simulink model "modello_prova_kalman_17_03"  (R2020b)
settings: Solver=VariableStepAuto  StartTime=0.0  StopTime=800  RelTol=1e-3
values from neighbouring files (symbols this model uses):
  bias = [baccxINI_new,baccyINI_new,bacczINI_new,bpINI_new,bqINI_new,brINI_new]    [Loader_HIL.m]
  Sensor_Offsets = [0,0,0]    [Loader_HIL.m]
  UP = 2    [Loader_HIL.m]
  vd_ini = 0    [Loader_HIL.m]
undefined symbols (not defined in the file or in its folder): Q1B, R1B, t_AP
libraries: simulink_extras x6, aerosimlib x2, cstblocks x1, dspsigops x1
settings Model: Creator=User  LastModifiedBy=SUSANNA

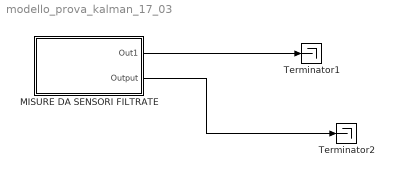
== system modello_prova_kalman_17_03 ==
  MISURE DA SENSORI FILTRATE : Subsystem
  Terminator1 : Terminator
  Terminator2 : Terminator
  wires:
  MISURE DA SENSORI FILTRATE/1(Out1) -> Terminator1/1
  MISURE DA SENSORI FILTRATE/2(Output) -> Terminator2/1

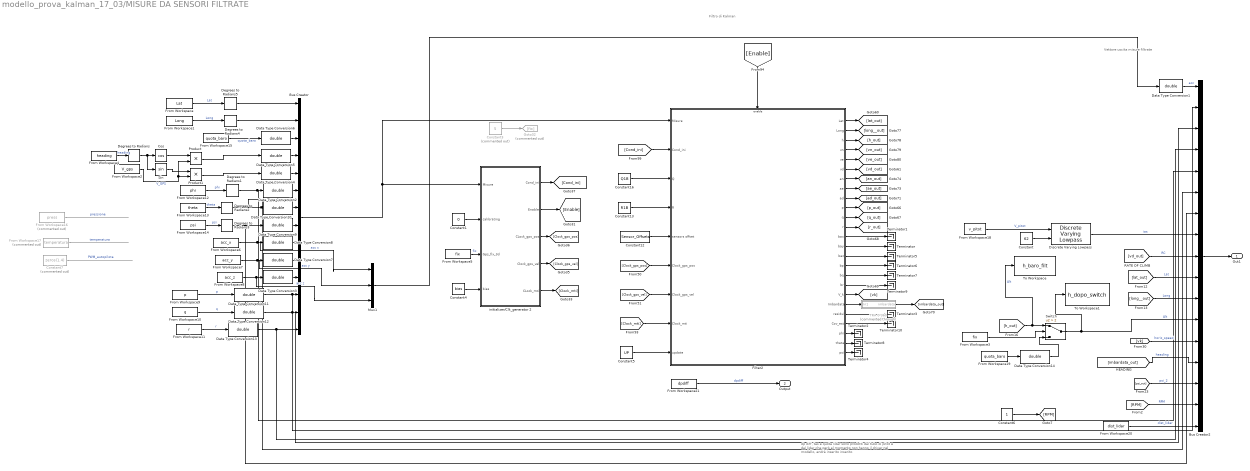
== system modello_prova_kalman_17_03/MISURE DA SENSORI FILTRATE ==
  note: dp diff, tas e quota lidar
      |  sono prodotti dal tubo di pitot e dal lidar che però al momento non hanno il driver nel modello, andrà inserito inserito
  note: Vettore uscita misure filtrate
  note: Filtro di Kalman
  Bus Creator : BusCreator  Inputs=14
  Bus Creator2 : BusCreator  Inputs=17
  Constant : Constant  Value=62
  Constant1 : Constant  Value=0
  Constant12 : Constant  Value=Sensor_Offsets
  Constant13 : Constant  Value=R1B
  Constant16 : Constant  Value=Q1B
  Constant3 : Constant  Commented=on  Value=5
  Constant4 : Constant  Value=bias
  Constant5 : Constant  Value=UP
  Constant6 : Constant
  Constant7 : Constant  Commented=on  Value=zeros(1,4)
  Cos : Trigonometry  Operator=cos
  Data Type Conversion{1..14} (14 alike) : DataTypeConversion  OutDataTypeStr=double
  Degrees to Radians{,1..5} (6 alike) : simulink_extras/Transformations/Degrees to Radians
  Discrete Varying Lowpass : cstblocks/Linear Parameter Varying/Discrete Varying Lowpass  N=1  w0=0  Ts=t_AP
      settings: SourceProductBaseCode=CT
  Filter2 : Subsystem
  From Workspace : FromWorkspace  VariableName=Lat  SampleTime=0.02
  From Workspace1 : FromWorkspace  VariableName=Long  SampleTime=0.02
  From Workspace10 : FromWorkspace  VariableName=q  SampleTime=0.02
  From Workspace11 : FromWorkspace  VariableName=r  SampleTime=0.02
  From Workspace12 : FromWorkspace  VariableName=phi  SampleTime=0.02
  From Workspace13 : FromWorkspace  VariableName=theta  SampleTime=0.02
  From Workspace14 : FromWorkspace  VariableName=psi  SampleTime=0.02
  From Workspace15 : FromWorkspace  VariableName=quota_baro
  From Workspace16 : FromWorkspace  Commented=on  VariableName=press
  From Workspace17 : FromWorkspace  Commented=on  VariableName=temperatura
  From Workspace18 : FromWorkspace  VariableName=v_pitot  SampleTime=0.02
  From Workspace19 : FromWorkspace  VariableName=quota_baro  SampleTime=0.02
  From Workspace2 : FromWorkspace  VariableName=V_gps  SampleTime=0.02
  From Workspace20 : FromWorkspace  VariableName=dist_lidar  SampleTime=0.02
  From Workspace21 : FromWorkspace  VariableName=dpdiff
  From Workspace3 : FromWorkspace  VariableName=fix  SampleTime=0.02
  From Workspace4 : FromWorkspace  VariableName=heading  SampleTime=0.02
  From Workspace5 : FromWorkspace  VariableName=fix
  From Workspace6 : FromWorkspace  VariableName=acc_x  SampleTime=0.02
  From Workspace7 : FromWorkspace  VariableName=acc_y  SampleTime=0.02
  From Workspace8 : FromWorkspace  VariableName=acc_z  SampleTime=0.02
  From Workspace9 : FromWorkspace  VariableName=p  SampleTime=0.02
  Goto32 : Goto  Commented=on  GotoTag=fix
  Mux1 : Mux  Inputs=3
  Product : Product
  Product1 : Product
  Sin : Trigonometry
  Switch : Switch  Criteria=u2 > Threshold  Threshold=2
  TRA 0-360 : Subsystem  Commented=through
  Terminator{,1..10} (11 alike) : Terminator
  To Workspace : ToWorkspace  VariableName=h_baro_filt  SaveFormat=Timeseries  SampleTime=-1
  To Workspace1 : ToWorkspace  VariableName=h_dopo_switch  SaveFormat=Timeseries  SampleTime=-1
  initializer/Clk_generator 2 : Subsystem
  Out1 : Outport  VectorParamsAs1DForOutWhenUnconnected=off
  Output : Outport  Port=2
  wires:
  From Workspace11/1 -> Data Type Conversion13/1  "r"
  [vd_out] -> Bus Creator2/9  "RC"
  From Workspace12/1 -> Degrees to Radians1/1  "phi"
  From Workspace9/1 -> Data Type Conversion11/1  "p"
  [vk] -> Bus Creator2/13  "horiz_speed"
  [imbardata_out] -> Bus Creator2/14  "heading"
  From Workspace10/1 -> Data Type Conversion12/1  "q"
  From Workspace13/1 -> Degrees to Radians2/1  "theta"
  Bus Creator2/1 -> Out1/1
  Discrete Varying Lowpass/1 -> Bus Creator2/8  "ias"
  [RPM] -> Bus Creator2/16  "RPM"
  Data Type Conversion1/1 -> Bus Creator2/1  "acc"
  Mux1/1 -> Data Type Conversion1/1
  From Workspace14/1 -> Degrees to Radians3/1  "psi"
  [long__out] -> Bus Creator2/11  "Long"
  [h_out] -> To Workspace/1, Switch/1  "Alt"
  [lat_out] -> Bus Creator2/10  "Lat"
  initializer/Clk_generator 2/5(CLock_mti) -> [Clock_mti]
  Constant3/1 -> Goto32/1
  initializer/Clk_generator 2/2(Enable) -> [Enable]
  Constant1/1 -> initializer/Clk_generator 2/2(calibrating)
  initializer/Clk_generator 2/3(CLock_gps_pos) -> [Clock_gps_pos]
  Filter2/3(h) -> [h_out]
  Constant4/1 -> initializer/Clk_generator 2/4(bias)
  Filter2/25(psi) -> Terminator4/1
  Filter2/6(vd) -> [vd_out]
  Constant13/1 -> Filter2/4(R)
  Filter2/10(p) -> [p_out]
  Filter2/18(br) -> Terminator9/1
  Filter2/23(phi) -> Terminator2/1
  Filter2/14(bay) -> Terminator/1
  [Cond_ini] -> Filter2/2(Cond_ini)
  Filter2/7(an) -> [an_out]
  Filter2/12(r) -> [r_out]
  initializer/Clk_generator 2/1(Cond_ini) -> [Cond_ini]
  Filter2/24(theta) -> Terminator8/1
  Filter2/11(q) -> [q_out]
  initializer/Clk_generator 2/4("Clock_gps_vel ") -> [Clock_gps_vel]
  Bus Creator/1 -> initializer/Clk_generator 2/1(Misure), Filter2/1(Misure)
  Filter2/2(Long) -> [long__out]
  Filter2/8(ae) -> [ae_out]
  Filter2/16(bp) -> Terminator6/1
  Filter2/9(ad) -> [ad_out]
  Filter2/4(vn) -> [vn_out]
  Constant16/1 -> Filter2/3(Q)
  Filter2/22(Cov_est) -> Terminator10/1
  Filter2/17(bq) -> Terminator7/1
  Filter2/21(residui) -> Terminator3/1
  [Clock_gps_vel] -> Filter2/7(Clock_gps_vel)
  Filter2/1(Lat) -> [lat_out]
  Filter2/15(baz) -> Terminator5/1
  [Enable] -> Filter2/Enable
  Filter2/19(V_k) -> [vk]
  Filter2/20(Imbardata) -> TRA 0-360/1(In1)
  Constant12/1 -> Filter2/5(sensors offset)
  Filter2/13(bax) -> Terminator1/1
  Filter2/5(ve) -> [ve_out]
  Constant5/1 -> Filter2/9(update)
  [Clock_gps_pos] -> Filter2/6(Clock_gps_pos)
  TRA 0-360/1(imbardata) -> [imbardata_out]
  [Clock_mti] -> Filter2/8(Clock_mti)
  Constant/1 -> Discrete Varying Lowpass/2
  Constant6/1 -> [RPM]
  [psi_out] -> Bus Creator2/15  "psi_2"
  From Workspace3/1 -> Switch/2
  From Workspace19/1 -> Data Type Conversion14/1
  Switch/1 -> To Workspace1/1, Bus Creator2/12  "Alt"
  From Workspace17/1 -> ?  "temperatura"
  From Workspace20/1 -> Bus Creator2/17  "dist_lidar"
  From Workspace/1 -> Degrees to Radians5/1  "Lat"
  From Workspace1/1 -> Degrees to Radians4/1  "Long"
  From Workspace18/1 -> Discrete Varying Lowpass/1  "V_pitot"
  From Workspace6/1 -> Mux1/1, Data Type Conversion8/1  "acc x"
  From Workspace8/1 -> Data Type Conversion3/1, Mux1/3  "acc z"
  From Workspace15/1 -> Data Type Conversion6/1  "quota_baro"
  Constant7/1 -> ?  "PWM_autopilota"
  From Workspace16/1 -> ?  "pressione"
  From Workspace21/1 -> Output/1  "dpdiff"
  From Workspace4/1 -> Degrees to Radians/1  "heading"
  From Workspace2/1 -> Product1/2, Product/2  "V_GPS"
  Sin/1 -> Product1/1
  Cos/1 -> Product/1
  Product/1 -> Data Type Conversion5/1
  Product1/1 -> Data Type Conversion4/1
  From Workspace7/1 -> Data Type Conversion7/1, Mux1/2  "acc y"
  From Workspace5/1 -> initializer/Clk_generator 2/3(Gps_fix_3d)  "fix"
  Degrees to Radians/1 -> Sin/1, Cos/1
  Degrees to Radians1/1 -> Bus Creator2/5, Data Type Conversion2/1
  Degrees to Radians2/1 -> Data Type Conversion10/1, Bus Creator2/6
  Degrees to Radians3/1 -> Bus Creator2/7, Data Type Conversion9/1
  Degrees to Radians4/1 -> Bus Creator/2
  Degrees to Radians5/1 -> Bus Creator/1
  Data Type Conversion6/1 -> Bus Creator/3
  Data Type Conversion5/1 -> Bus Creator/4
  Data Type Conversion4/1 -> Bus Creator/5
  Data Type Conversion2/1 -> Bus Creator/6
  Data Type Conversion10/1 -> Bus Creator/7
  Data Type Conversion9/1 -> Bus Creator/8
  Data Type Conversion8/1 -> Bus Creator/9
  Data Type Conversion7/1 -> Bus Creator/10
  Data Type Conversion3/1 -> Bus Creator/11
  Data Type Conversion11/1 -> Bus Creator2/2, Bus Creator/12
  Data Type Conversion12/1 -> Bus Creator2/3, Bus Creator/13
  Data Type Conversion13/1 -> Bus Creator2/4, Bus Creator/14
  Data Type Conversion14/1 -> Switch/3

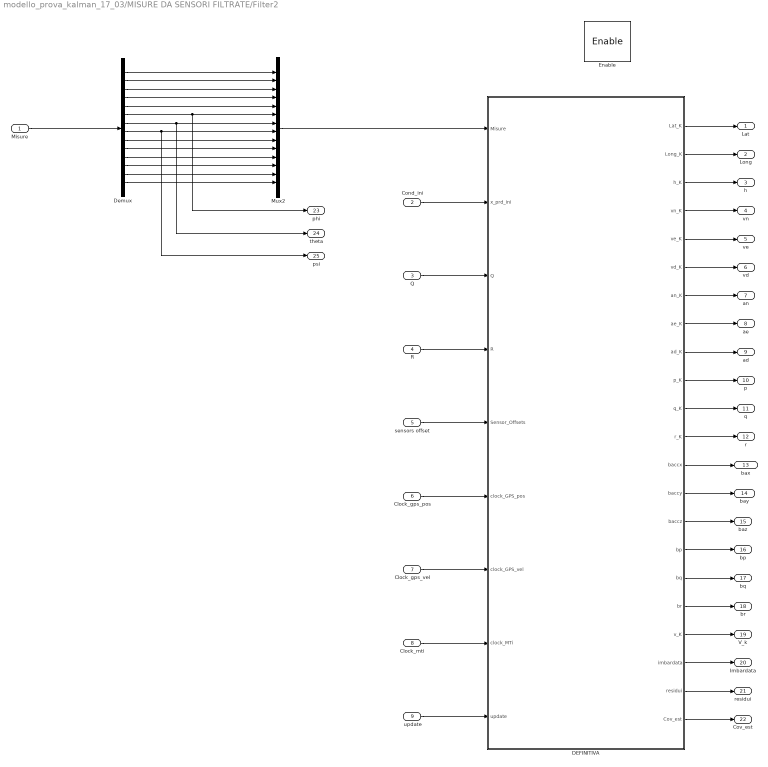
== system modello_prova_kalman_17_03/MISURE DA SENSORI FILTRATE/Filter2 ==
  Misure : Inport
  Cond_ini : Inport  Port=2
  Q : Inport  Port=3
  R : Inport  Port=4
  sensors offset : Inport  Port=5
  Clock_gps_pos : Inport  Port=6
  Clock_gps_vel : Inport  Port=7
  Clock_mti : Inport  Port=8
  update : Inport  Port=9
  Enable : EnablePort
  DEFINITIVA : MATLAB Function  TreatAsAtomicUnit=on
  Demux : Demux  Outputs=14
  Mux2 : Mux  Inputs=14
  Lat : Outport  VectorParamsAs1DForOutWhenUnconnected=off
  Long : Outport  Port=2  VectorParamsAs1DForOutWhenUnconnected=off
  h : Outport  Port=3  VectorParamsAs1DForOutWhenUnconnected=off
  vn : Outport  Port=4  VectorParamsAs1DForOutWhenUnconnected=off
  ve : Outport  Port=5  VectorParamsAs1DForOutWhenUnconnected=off
  vd : Outport  Port=6  VectorParamsAs1DForOutWhenUnconnected=off
  an : Outport  Port=7  VectorParamsAs1DForOutWhenUnconnected=off
  ae : Outport  Port=8  VectorParamsAs1DForOutWhenUnconnected=off
  ad : Outport  Port=9  VectorParamsAs1DForOutWhenUnconnected=off
  p : Outport  Port=10  VectorParamsAs1DForOutWhenUnconnected=off
  q : Outport  Port=11  VectorParamsAs1DForOutWhenUnconnected=off
  r : Outport  Port=12  VectorParamsAs1DForOutWhenUnconnected=off
  bax : Outport  Port=13  VectorParamsAs1DForOutWhenUnconnected=off
  bay : Outport  Port=14  VectorParamsAs1DForOutWhenUnconnected=off
  baz : Outport  Port=15  VectorParamsAs1DForOutWhenUnconnected=off
  bp : Outport  Port=16  VectorParamsAs1DForOutWhenUnconnected=off
  bq : Outport  Port=17  VectorParamsAs1DForOutWhenUnconnected=off
  br : Outport  Port=18  VectorParamsAs1DForOutWhenUnconnected=off
  V_k : Outport  Port=19  VectorParamsAs1DForOutWhenUnconnected=off
  Imbardata : Outport  Port=20  VectorParamsAs1DForOutWhenUnconnected=off
  residui : Outport  Port=21  VectorParamsAs1DForOutWhenUnconnected=off
  Cov_est : Outport  Port=22  VectorParamsAs1DForOutWhenUnconnected=off
  phi : Outport  Port=23  VectorParamsAs1DForOutWhenUnconnected=off
  theta : Outport  Port=24  VectorParamsAs1DForOutWhenUnconnected=off
  psi : Outport  Port=25  VectorParamsAs1DForOutWhenUnconnected=off
  wires:
  Misure/1 -> Demux/1
  Demux/10 -> Mux2/10
  Demux/13 -> Mux2/13
  Demux/11 -> Mux2/11
  Demux/4 -> Mux2/4
  Demux/14 -> Mux2/14
  Demux/7 -> theta/1, Mux2/7
  Demux/12 -> Mux2/12
  Demux/6 -> phi/1, Mux2/6
  Demux/5 -> Mux2/5
  Demux/9 -> Mux2/9
  Demux/8 -> psi/1, Mux2/8
  Demux/3 -> Mux2/3
  DEFINITIVA/8(ae_K) -> ae/1
  DEFINITIVA/7(an_K) -> an/1
  DEFINITIVA/11(q_K) -> q/1
  DEFINITIVA/2(Long_K) -> Long/1
  DEFINITIVA/3(h_K) -> h/1
  DEFINITIVA/10(p_K) -> p/1
  DEFINITIVA/6(vd_K) -> vd/1
  DEFINITIVA/13(baccx) -> bax/1
  DEFINITIVA/20(imbardata) -> Imbardata/1
  DEFINITIVA/19(v_K) -> V_k/1
  DEFINITIVA/18(br) -> br/1
  DEFINITIVA/4(vn_K) -> vn/1
  DEFINITIVA/16(bp) -> bp/1
  DEFINITIVA/21(residui) -> residui/1
  DEFINITIVA/17(bq) -> bq/1
  DEFINITIVA/5(ve_K) -> ve/1
  DEFINITIVA/12(r_K) -> r/1
  DEFINITIVA/1(Lat_K) -> Lat/1
  DEFINITIVA/22(Cov_est) -> Cov_est/1
  DEFINITIVA/15(baccz) -> baz/1
  DEFINITIVA/14(baccy) -> bay/1
  DEFINITIVA/9(ad_K) -> ad/1
  Mux2/1 -> DEFINITIVA/1(Misure)
  Cond_ini/1 -> DEFINITIVA/2(x_prd_ini)
  Q/1 -> DEFINITIVA/3(Q)
  R/1 -> DEFINITIVA/4(R)
  sensors offset/1 -> DEFINITIVA/5(Sensor_Offsets)
  Clock_gps_pos/1 -> DEFINITIVA/6(clock_GPS_pos)
  Clock_gps_vel/1 -> DEFINITIVA/7(clock_GPS_vel)
  Clock_mti/1 -> DEFINITIVA/8(clock_MTi)
  update/1 -> DEFINITIVA/9(update)
  Demux/2 -> Mux2/2
  Demux/1 -> Mux2/1

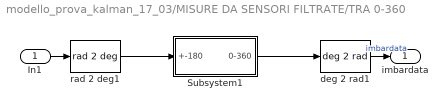
== system modello_prova_kalman_17_03/MISURE DA SENSORI FILTRATE/TRA 0-360 ==
  In1 : Inport
  Subsystem1 : Subsystem
  deg 2 rad1 : aerosimlib/Unit Conversion/Angular position/deg 2 rad
      settings: SourceProductName=AeroSim Blockset
  rad 2 deg1 : aerosimlib/Unit Conversion/Angular position/rad 2 deg
      settings: SourceProductName=AeroSim Blockset
  imbardata : Outport  VectorParamsAs1DForOutWhenUnconnected=off
  wires:
  deg 2 rad1/1 -> imbardata/1  "imbardata"
  rad 2 deg1/1 -> Subsystem1/1(+-180)
  In1/1 -> rad 2 deg1/1
  Subsystem1/1(0-360) -> deg 2 rad1/1

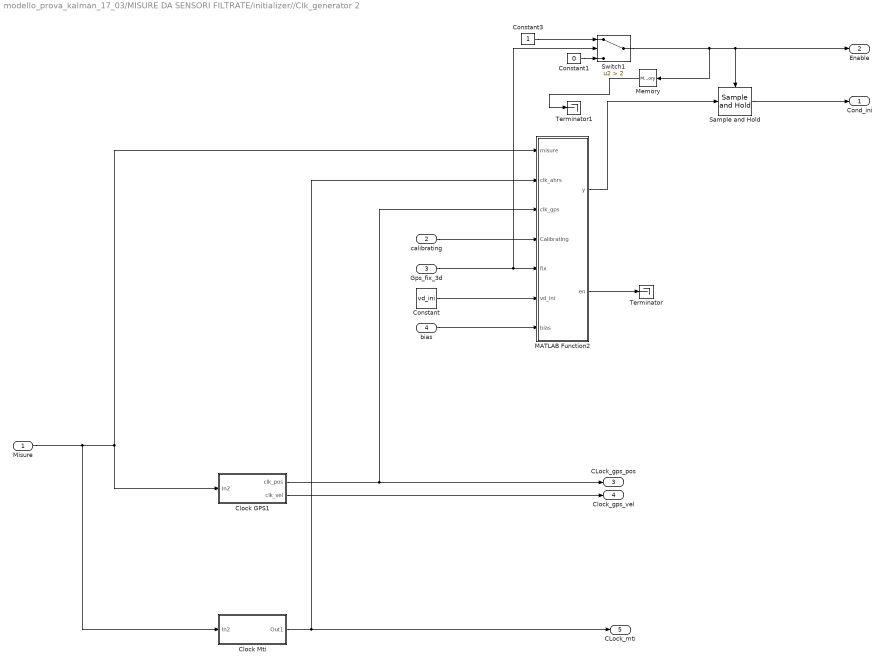
== system modello_prova_kalman_17_03/MISURE DA SENSORI FILTRATE/initializer//Clk_generator 2 ==
  Misure : Inport
  calibrating : Inport  Port=2
  Gps_fix_3d : Inport  Port=3
  bias : Inport  Port=4
  Clock GPS1 : Subsystem
  Clock Mti : Subsystem
  Constant : Constant  Value=vd_ini
  Constant1 : Constant  Value=0
  Constant3 : Constant
  MATLAB Function2 : MATLAB Function  TreatAsAtomicUnit=on
  Memory : Memory  InheritSampleTime=on
  Sample and Hold : dspsigops/Sample and Hold  trig=Rising edge  initCond=0  latchinput=off
  Switch1 : Switch  Criteria=u2 > Threshold  Threshold=2
  Terminator : Terminator
  Terminator1 : Terminator
  Cond_ini : Outport  VectorParamsAs1DForOutWhenUnconnected=off
  Enable : Outport  Port=2  VectorParamsAs1DForOutWhenUnconnected=off
  CLock_gps_pos : Outport  Port=3  VectorParamsAs1DForOutWhenUnconnected=off
  "Clock_gps_vel " : Outport  Port=4  VectorParamsAs1DForOutWhenUnconnected=off
  CLock_mti : Outport  Port=5  VectorParamsAs1DForOutWhenUnconnected=off
  wires:
  Clock GPS1/1(clk_pos) -> MATLAB Function2/3(clk_gps), CLock_gps_pos/1
  Clock Mti/1(Out1) -> CLock_mti/1, MATLAB Function2/2(clk_ahrs)
  Constant/1 -> MATLAB Function2/6(vd_ini)
  bias/1 -> MATLAB Function2/7(bias)
  calibrating/1 -> MATLAB Function2/4(Calibrating)
  Misure/1 -> Clock Mti/1(In2), Clock GPS1/1(In2), MATLAB Function2/1(misure)
  Clock GPS1/2(clk_vel) -> "Clock_gps_vel "/1
  MATLAB Function2/1(y) -> Sample and Hold/1
  Sample and Hold/1 -> Cond_ini/1
  MATLAB Function2/2(en) -> Terminator/1
  Gps_fix_3d/1 -> Switch1/2, MATLAB Function2/5(fix)
  Switch1/1 -> Memory/1, Enable/1, Sample and Hold/Trigger
  Constant3/1 -> Switch1/1
  Memory/1 -> Terminator1/1
  Constant1/1 -> Switch1/3

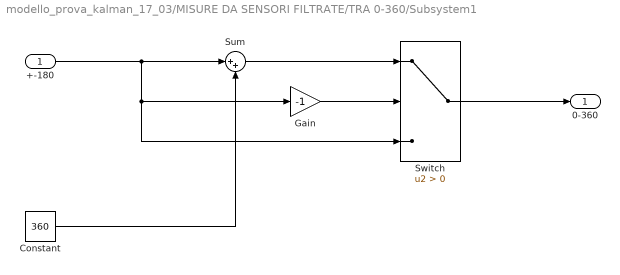
== system modello_prova_kalman_17_03/MISURE DA SENSORI FILTRATE/TRA 0-360/Subsystem1 ==
  +-180 : Inport
  Constant : Constant  Value=360
  Gain : Gain  Gain=-1
  Sum : Sum  Inputs=|++
  Switch : Switch  Criteria=u2 > Threshold
  0-360 : Outport  VectorParamsAs1DForOutWhenUnconnected=off
  wires:
  Constant/1 -> Sum/2
  +-180/1 -> Gain/1, Switch/3, Sum/1
  Gain/1 -> Switch/2
  Sum/1 -> Switch/1
  Switch/1 -> 0-360/1

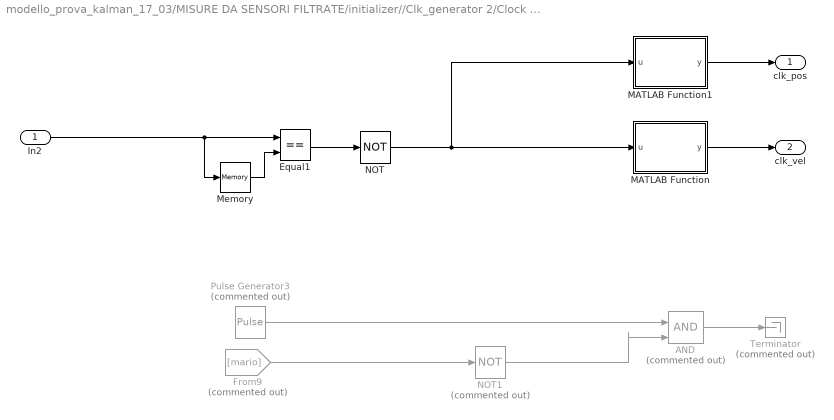
== system modello_prova_kalman_17_03/MISURE DA SENSORI FILTRATE/initializer//Clk_generator 2/Clock GPS1 ==
  In2 : Inport
  AND : Logic  Commented=on  IconShape=distinctive  AllPortsSameDT=off  OutDataTypeStr=boolean
  Equal1 : RelationalOperator  Operator===  OutDataTypeStr=boolean  RndMeth=Simplest
  From9 : From  Commented=on  GotoTag=mario
  MATLAB Function : MATLAB Function  TreatAsAtomicUnit=on
  MATLAB Function1 : MATLAB Function  TreatAsAtomicUnit=on
  Memory : Memory
  NOT : Logic  Operator=NOT  IconShape=distinctive  AllPortsSameDT=off  OutDataTypeStr=boolean
  NOT1 : Logic  Commented=on  Operator=NOT  IconShape=distinctive  AllPortsSameDT=off  OutDataTypeStr=boolean
  Pulse Generator3 : DiscretePulseGenerator  Commented=on  PulseType=Time based  Period=0.2  PulseWidth=10
  Terminator : Terminator  Commented=on
  clk_pos : Outport  VectorParamsAs1DForOutWhenUnconnected=off
  clk_vel : Outport  Port=2  VectorParamsAs1DForOutWhenUnconnected=off
  wires:
  Equal1/1 -> NOT/1
  NOT/1 -> MATLAB Function1/1(u), MATLAB Function/1(u)
  In2/1 -> Equal1/1, Memory/1
  Memory/1 -> Equal1/2
  From9/1 -> NOT1/1
  Pulse Generator3/1 -> AND/1
  NOT1/1 -> AND/2
  AND/1 -> Terminator/1
  MATLAB Function1/1(y) -> clk_pos/1
  MATLAB Function/1(y) -> clk_vel/1

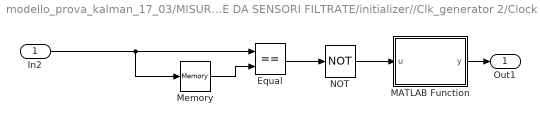
== system modello_prova_kalman_17_03/MISURE DA SENSORI FILTRATE/initializer//Clk_generator 2/Clock Mti ==
  In2 : Inport
  Equal : RelationalOperator  Operator===  OutDataTypeStr=boolean  RndMeth=Simplest
  MATLAB Function : MATLAB Function  TreatAsAtomicUnit=on
  Memory : Memory
  NOT : Logic  Operator=NOT  IconShape=distinctive  AllPortsSameDT=off  OutDataTypeStr=boolean
  Out1 : Outport  VectorParamsAs1DForOutWhenUnconnected=off
  wires:
  In2/1 -> Memory/1, Equal/1
  Equal/1 -> NOT/1
  Memory/1 -> Equal/2
  MATLAB Function/1(y) -> Out1/1
  NOT/1 -> MATLAB Function/1(u)

== matlab function modello_prova_kalman_17_03/MISURE DA SENSORI FILTRATE/Filter2/DEFINITIVA ==
  settings: updateMethod=DISCRETE  sampleTime=0.02
  data: Lat_K output; Misure input; x_prd_ini input; Q input; R input; Sensor_Offsets input; clock_GPS_pos input; clock_GPS_vel input; clock_MTi input; Long_K output; h_K output; vn_K output; ve_K output; vd_K output; an_K output; ae_K output; ad_K output; p_K output; q_K output; r_K output; baccx output; baccy output; baccz output; bp output; bq output; br output; v_K output; imbardata output; residui output; update input; Cov_est output
function [Lat_K,Long_K,h_K,vn_K,ve_K,vd_K,an_K,ae_K,ad_K,p_K,q_K,r_K,baccx,baccy,baccz,bp,bq,br,v_K,imbardata,residui,Cov_est]     = FILTRO_1B(Misure,x_prd_ini,Q,R,Sensor_Offsets,clock_GPS_pos,clock_GPS_vel,clock_MTi,update)

persistent x_prd
persistent p_prd 

%% Parametri

a = 6378137; % earth radius (m)
g = 9.81;      % gravity constant (m/s^2)
Misure(1)=cast(Misure(1),'double');
Misure(2)=cast(Misure(2),'double');
Z = Misure;
EULERO=[Z(6),Z(7),Z(8)];
% Z(9)=-Misure(9);

  infinito = 1e40;

dt=0.02; %sample time

%      Sensor Offsets     %% Da spostere in avvio simulazione

rx = Sensor_Offsets(1);

ry = Sensor_Offsets(2);

rz =Sensor_Offsets(3);

% Inizializzo stato e covarianza

% if isempty(x_prd)
%    
%     x_prd = x_prd_ini;
% 
%  	p_prd =zeros(18,18);
%     
% end




if isempty(x_prd)
   x_prd=zeros(1,18);
   
     x_prd(1) = x_prd_ini(1); %Posizione 
     x_prd(2) = x_prd_ini(2);
     x_prd(3) = x_prd_ini(3);
     
     x_prd(4) = x_prd_ini(4); %Velocità
     x_prd(5) = x_prd_ini(5);
     x_prd(6) = x_prd_ini(6); 
     
     x_prd(7) = x_prd_ini(10); %Acc
     x_prd(8) = x_prd_ini(11);
     x_prd(9)= x_prd_ini(12);
     
     x_prd(10) = x_prd_ini(13); %V ang
     x_prd(11) = x_prd_ini(14);
     x_prd(12)=  x_prd_ini(15);
     
     x_prd(13) = x_prd_ini(16); %Bias Acc
     x_prd(14) = x_prd_ini(17);
     x_prd(15)=  x_prd_ini(18);
     
     x_prd(16) = x_prd_ini(19); %Bias Vang
     x_prd(17) = x_prd_ini(20);
     x_prd(18)=  x_prd_ini(21);
     
%  	p_prd =10000*eye(18,18);
      p_prd =zeros(18,18);
      p_prd(1,1)=10000000000;
      p_prd(4,4)=10000000000;
      p_prd(5,5)=10000000000;
end

%%%%%%%%%%%%%%%%%%%%%%%%%%%
%% Predicted measurement %%  
%calcolo della stima a priori dello stato x al passo k condizionata dai passi
%precedenti fino a k-1 ovvero x(k|k-1) (partendo dal presupposto di conoscere la previsione
% dello stato x(k-1|jk-1) che tiene conto anche delle misure)
%%SONO LE EQUAZIONI DELLE EVOLUZIONI DELLE MISURE


Y_prd = measure_F1B(x_prd,EULERO,rx,ry,rz,g);


%%%%%%%%%%%%%%%%%%%%%%%%%%%
%% Linearize measurement-jacobiano delle equazioni delle misure%%
%%%%%%%%%%%%%%%%%%%%%%%%%%%

H=jac_H_F1B(x_prd,EULERO,rx,ry,rz,g);


%%%%%%%%%%%%%%%%%%%%%%%%  
%% aggiornamento della misura %%

%per la matrice covarianza dell'errore di stima dello stato che è definita
%come P(k|k)=P(k|k-1)-K(k)H(k)S(k)^-1 con S(k)=H(k)P(k|k-1)H(k)+R(k)
%con P(k|k-1) definibile dalla dtima a priori, R(k) è il valore atteso del
%vettore del rumore delle misure e K(k) è il guadagno di kalman
%%%%%%%%%%%%%%%%%%%%%%%%

% Estimation of measurement

S = H *p_prd* H.';

%%

switch update
    case 0
        
        for i = 1:11
    S(i,i) = S(i,i) + R(i); %%%%%
        end
        
    case 1
        
        if clock_GPS_pos == 0 
for i = 1:11               
        if i == 1 || i == 2      
            S(i,i) = S(i,i) +infinito;     
        else            
            S(i,i) = S(i,i) + R(i);              
        end          
end 

else 
    for i = 1:11
    S(i,i) = S(i,i) + R(i); %%%%%
    end
        end

    case 2
        
        if clock_GPS_pos == 1 && clock_GPS_vel == 1  && clock_MTi == 1
    
    for i = 1:11
        
        S(i,i) = S(i,i) + R(i);
       
    end
		 
elseif clock_GPS_pos == 0 && clock_GPS_vel == 1 && clock_MTi == 1 
    
    for i = 1:11                
        if i == 1 || i == 2               
            S(i,i) = S(i,i) +infinito;     
        else            
            S(i,i) = S(i,i) + R(i);              
        end          
    end
    
elseif clock_GPS_pos == 1 && clock_GPS_vel == 0 && clock_MTi == 1 
    
    for i = 1:11                
        if i == 4 || i == 5               
            S(i,i) = S(i,i) +infinito;     
        else            
            S(i,i) = S(i,i) + R(i);              
        end          
    end
    
   elseif clock_GPS_pos == 0 && clock_GPS_vel == 0 && clock_MTi == 1 
    
    for i = 1:11                
        if i == 1 || i == 2 || i == 4 || i == 5               
            S(i,i) = S(i,i) +infinito;     
        else            
            S(i,i) = S(i,i) + R(i);              
        end          
    end
    %
     
    
    elseif clock_GPS_pos == 1 && clock_GPS_vel == 1  && clock_MTi == 0
    
    for i = 1:11

        if i == 1 || i == 2 || i == 4 || i == 5 || i == 3              

        S(i,i) = S(i,i) +R(i);
        else
        S(i,i) = S(i,i) +infinito;     
  
        end 
    end
		 
elseif clock_GPS_pos == 0 && clock_GPS_vel == 1 && clock_MTi == 0
    
    for i = 1:11          
        
        if i == 4 || i == 5 || i == 3              

        S(i,i) = S(i,i) +R(i);
        else
        S(i,i) = S(i,i) +infinito;     
  
        end   
    end
    
elseif clock_GPS_pos == 1 && clock_GPS_vel == 0 && clock_MTi == 0 
    
    for i = 1:11               
        if i == 1 || i == 2 || i == 3              

        S(i,i) = S(i,i) +R(i);
        else
        S(i,i) = S(i,i) +infinito;     
  
        end           
    end
    
   elseif clock_GPS_pos == 0 && clock_GPS_vel == 0 && clock_MTi == 0 
    
    for i = 1:11                 
         if  i == 3              
         S(i,i) = S(i,i) +R(i);
        else
        S(i,i) = S(i,i) +infinito;     
  
        end                     
    end 
    
end
end



C = H * p_prd.'; 

klm_gain = (S \ C).';


Z_=zeros(11,1);

Z_(1)= Z(1);  %Pos
Z_(2)= Z(2);
Z_(3)= Z(3);

Z_(4)= Z(4);   %Vel
Z_(5)= Z(5);

Z_(6)= Z(9);   %acc
Z_(7)= Z(10);
Z_(8)= Z(11);

Z_(9)= Z(12);   %vel ang
Z_(10)= Z(13);
Z_(11)= Z(14);

errore_prd = (Z_ - Y_prd); % 




residui = errore_prd;

x_est = x_prd + (klm_gain * (errore_prd)).';
p_est = p_prd - klm_gain * H * p_prd;

Cov_est=diag(p_est);

    % K_gain=zeros(21,1);
% 
% for i=1:21
%     
%    K_gain(i)=klm_gain(i,i);
%    
% end

%%%%%%%%%%%%%%%%%%%%%%%%
%% linearizzazione dinamica-jacobiano delle equazioni di evoluzione di stato
%%%%%%%%%%%%%%%%%%%%%%%%

F = jac_F_F1B(x_est,a,dt);

%%%%%%%%%%%%%%%%%                                            
%% aggiornamento con le equazioni della evoluzione di stato %%
%%%%%%%%%%%%%%%%%


x_prd = (f_pred_F1B(x_est,a,dt)).';



% Predicted covariance update

p_prd = F * p_est * F.';

for k = 1:18
    
    p_prd(k,k) = p_prd(k,k) + Q(k);
    
end

%%%%%%%%%%
%% Exit %%
%%%%%%%%%%  

Lat_K = x_est(1);
Long_K = x_est(2);
h_K = x_est(3);

vn_K = x_est(4);
ve_K = x_est(5);
vd_K = x_est(6);


% phi_K = x_est(7);
% theta_K = x_est(8);
% psi_K = x_est(9);

an_K = x_est(7);
ae_K = x_est(8);
ad_K = x_est(9);


p_K = x_est(10);
q_K = x_est(11);
r_K = x_est(12);

baccx = x_est(13);
baccy = x_est(14);
baccz = x_est(15);

bp = x_est(16);
bq = x_est(17);
br = x_est(18);

imbardata = atan2(ve_K,vn_K);
v_K = sqrt(vn_K^2 + ve_K^2);

== matlab function modello_prova_kalman_17_03/MISURE DA SENSORI FILTRATE/initializer//Clk_generator 2/Clock GPS1/MATLAB Function ==
  data: u input; y output
function y = fcn(u)

 y = u(4) || u(5);

% if mario ~=0
%     
%     y=double(0);
%     
% else 
%      y = u(1) || u(2) || u(3) || u(4);
% 
%  end

== matlab function modello_prova_kalman_17_03/MISURE DA SENSORI FILTRATE/initializer//Clk_generator 2/Clock GPS1/MATLAB Function1 ==
  data: u input; y output
function y = fcn(u)

 y = u(1) || u(2);
% if mario ~=0
%     
%     y=double(0);
%     
% else 
%      y = u(1) || u(2) || u(3) || u(4);
% 
%  end

== matlab function modello_prova_kalman_17_03/MISURE DA SENSORI FILTRATE/initializer//Clk_generator 2/Clock Mti/MATLAB Function ==
  data: u input; y output
function y = fcn(u)

y = u(6)|| u(7)|| u(8)||  u(9) || u(10)|| u(11) || u(12) || u(13);

== matlab function modello_prova_kalman_17_03/MISURE DA SENSORI FILTRATE/initializer//Clk_generator 2/MATLAB Function2 ==
  data: misure input; clk_ahrs input; y output; clk_gps input; Calibrating input; en output; fix input; vd_ini input; bias input
function [y,en] = fcn(misure,clk_ahrs,clk_gps,Calibrating, fix,vd_ini, bias)

    
     y=zeros(21,1);
    
     phi = misure(6);
     theta = misure(7);
     psi = misure(8);
    
     ab=[misure(9);misure(10);misure(11)];
     
     
    LBE= [cos(psi)*cos(theta) ,cos(psi)*sin(phi)*sin(theta)-cos(phi)*sin(psi) ,cos(phi)*cos(psi)*sin(theta)+sin(phi)*sin(psi);
    
      sin(psi)*cos(theta) ,sin(phi)*sin(psi)*sin(theta)+cos(phi)*cos(psi) , cos(phi)*sin(psi)*sin(theta)-cos(psi)*sin(phi);
      
      -sin(theta),cos(theta)*sin(phi),cos(phi)*cos(theta)];
      
      aterra=LBE*ab;
   
    
    y(1) = misure(1);
    y(2) = misure(2);
    y(3) = misure(3);
    
    
    y(4) = misure(4);
    y(5) = misure(5);
    y(6) = vd_ini;
    
    y(7) = misure(6);
    y(8) = misure(7);
    y(9) = misure(8);
    
    y(10) = aterra(1);
    y(11) = aterra(2);
    y(12) = aterra(3);
    
    y(13) = misure(12);
    y(14) = misure(13);
    y(15) = misure(14);
    
    y(16) = bias(1);
    y(17) = bias(2);
    y(18) = bias(3);
    
    y(19) = bias(4);
    y(20) = bias(5);
    y(21) = bias(6);
    
    
en=1;
